simulink model "batt"  (R2018b)
settings: Solver=VariableStepAuto  StartTime=0.0  StopTime=3600  RelTol=1e-3
undefined symbols (not defined in the file or in its folder): Batt
settings Model: Creator=Pedro  LastModifiedBy=Pedro

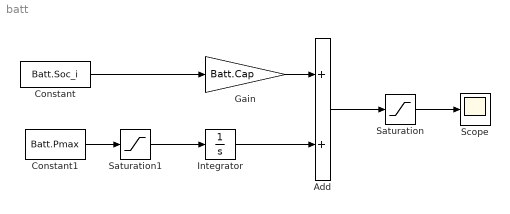
== system batt ==
  Add : Sum
  Constant : Constant  Value=Batt.Soc_i
  Constant1 : Constant  Value=Batt.Pmax
  Gain : Gain  Gain=Batt.Cap
  Integrator : Integrator
  Saturation : Saturate  UpperLimit=Batt.Cap  LowerLimit=0
  Saturation1 : Saturate  UpperLimit=Batt.Pmax  LowerLimit=-Batt.Pmax
  Scope : Scope
  wires:
  Constant1/1 -> Saturation1/1
  Saturation1/1 -> Integrator/1
  Add/1 -> Saturation/1
  Gain/1 -> Add/1
  Constant/1 -> Gain/1
  Saturation/1 -> Scope/1
  Integrator/1 -> Add/2
